simulink library "DAVS_lib"  (R2022b)
settings: Solver=VariableStepAuto  StartTime=0.0  StopTime=10.0  RelTol=1e-3
undefined symbols (not defined in the file): c0_ne, c0_pe, c_max_ne, c_max_pe, D_ne, D_pe, F, k, N_a_ne, N_a_pe, R_ne, R_pe
libraries: fl_lib x60, nesl_utility x60
(part 2 of 2)

== system DAVS_lib/DAVS/c_surf_ne/V(3)1/c(3) ==
  I(3) : Inport
  n : Inport  Port=2
  Divide : Product  Inputs=*/
  Gain : Gain  Gain=F
  Integrator : Integrator  InitialCondition=c0_ne
  Subsystem1 : Subsystem
  c(3) : Outport
  wires:
  Subsystem1/1(dV(n)1) -> Gain/1
  n/1 -> Subsystem1/1(n1)
  Integrator/1 -> c(3)/1
  Divide/1 -> Integrator/1
  Gain/1 -> Divide/2
  I(3)/1 -> Divide/1

== system DAVS_lib/DAVS/c_surf_ne/V(4)1/I(4) ==
  I_bar(3) : Inport
  I_bar(4) : Inport  Port=2
  Sum : Sum  Inputs=|-+|
  I(4) : Outport
  wires:
  I_bar(4)/1 -> Sum/1
  I_bar(3)/1 -> Sum/2
  Sum/1 -> I(4)/1

== system DAVS_lib/DAVS/c_surf_ne/V(4)1/Subsystem1 ==
  n : Inport
  Constant : Constant  Value=2
  Constant1 : Constant  Value=10
  Divide : Product  Inputs=*/
  Gain : Gain  Gain=k
  Gain1 : Gain  Gain=4*pi*R_ne*D_ne
  Math Function : Math  Operator=pow
  Rd : Outport
  wires:
  Constant1/1 -> Gain/1
  Divide/1 -> Rd/1
  Math Function/1 -> Gain1/1
  Gain1/1 -> Divide/2
  Constant/1 -> Math Function/2
  Gain/1 -> Divide/1
  n/1 -> Math Function/1

== system DAVS_lib/DAVS/c_surf_ne/V(4)1/V(4) ==
  c(4) : Inport
  Gain : Gain  Gain=k*F
  V(4) : Outport
  wires:
  c(4)/1 -> Gain/1
  Gain/1 -> V(4)/1

== system DAVS_lib/DAVS/c_surf_ne/V(4)1/c(4) ==
  I(4) : Inport
  n : Inport  Port=2
  Divide : Product  Inputs=*/
  Gain : Gain  Gain=F
  Integrator : Integrator  InitialCondition=c0_ne
  Subsystem1 : Subsystem
  c(4) : Outport
  wires:
  Subsystem1/1(dV(n)1) -> Gain/1
  n/1 -> Subsystem1/1(n1)
  I(4)/1 -> Divide/1
  Gain/1 -> Divide/2
  Divide/1 -> Integrator/1
  Integrator/1 -> c(4)/1

== system DAVS_lib/DAVS/c_surf_ne/V(5)1/I(n) ==
  I_bar(4) : Inport
  I_bar(5) : Inport  Port=2
  Sum : Sum  Inputs=|-+|
  I(5) : Outport
  wires:
  Sum/1 -> I(5)/1
  I_bar(4)/1 -> Sum/2
  I_bar(5)/1 -> Sum/1

== system DAVS_lib/DAVS/c_surf_ne/V(5)1/Subsystem1 ==
  n : Inport
  Constant : Constant  Value=2
  Constant1 : Constant  Value=10
  Divide : Product  Inputs=*/
  Gain : Gain  Gain=k
  Gain1 : Gain  Gain=4*pi*R_ne*D_ne
  Math Function : Math  Operator=pow
  Rd : Outport
  wires:
  Constant1/1 -> Gain/1
  Divide/1 -> Rd/1
  Math Function/1 -> Gain1/1
  Gain1/1 -> Divide/2
  Constant/1 -> Math Function/2
  Gain/1 -> Divide/1
  n/1 -> Math Function/1

== system DAVS_lib/DAVS/c_surf_ne/V(5)1/V(5) ==
  c(5) : Inport
  Gain : Gain  Gain=k*F
  V(5) : Outport
  wires:
  Gain/1 -> V(5)/1
  c(5)/1 -> Gain/1

== system DAVS_lib/DAVS/c_surf_ne/V(5)1/c(5) ==
  I(5) : Inport
  n : Inport  Port=2
  Divide : Product  Inputs=*/
  Gain : Gain  Gain=F
  Integrator : Integrator  InitialCondition=c0_ne
  Subsystem1 : Subsystem
  c(5) : Outport
  wires:
  Subsystem1/1(dV(n)1) -> Gain/1
  n/1 -> Subsystem1/1(n1)
  Integrator/1 -> c(5)/1
  Divide/1 -> Integrator/1
  Gain/1 -> Divide/2
  I(5)/1 -> Divide/1

== system DAVS_lib/DAVS/c_surf_ne/V(6)1/I(6) ==
  I_bar(6) : Inport
  I_bar(5) : Inport  Port=2
  Sum : Sum  Inputs=|-+|
  I(6) : Outport
  wires:
  I_bar(5)/1 -> Sum/1
  I_bar(6)/1 -> Sum/2
  Sum/1 -> I(6)/1

== system DAVS_lib/DAVS/c_surf_ne/V(6)1/Subsystem1 ==
  n : Inport
  Constant : Constant  Value=2
  Constant1 : Constant  Value=10
  Divide : Product  Inputs=*/
  Gain : Gain  Gain=k
  Gain1 : Gain  Gain=4*pi*R_ne*D_ne
  Math Function : Math  Operator=pow
  Rd : Outport
  wires:
  Constant1/1 -> Gain/1
  Divide/1 -> Rd/1
  Math Function/1 -> Gain1/1
  Gain1/1 -> Divide/2
  Constant/1 -> Math Function/2
  Gain/1 -> Divide/1
  n/1 -> Math Function/1

== system DAVS_lib/DAVS/c_surf_ne/V(6)1/V(6) ==
  c(6) : Inport
  Gain : Gain  Gain=k*F
  V(6) : Outport
  wires:
  c(6)/1 -> Gain/1
  Gain/1 -> V(6)/1

== system DAVS_lib/DAVS/c_surf_ne/V(6)1/c(6) ==
  I(6) : Inport
  n : Inport  Port=2
  Divide : Product  Inputs=*/
  Gain : Gain  Gain=F
  Integrator : Integrator  InitialCondition=c0_ne
  Subsystem1 : Subsystem
  c(6) : Outport
  wires:
  n/1 -> Subsystem1/1(n1)
  Subsystem1/1(dV(n)1) -> Gain/1
  I(6)/1 -> Divide/1
  Gain/1 -> Divide/2
  Divide/1 -> Integrator/1
  Integrator/1 -> c(6)/1

== system DAVS_lib/DAVS/c_surf_ne/V(7)1/I(7) ==
  I_bar(6) : Inport
  I_bar(7) : Inport  Port=2
  Sum : Sum  Inputs=|-+|
  I(7) : Outport
  wires:
  Sum/1 -> I(7)/1
  I_bar(6)/1 -> Sum/2
  I_bar(7)/1 -> Sum/1

== system DAVS_lib/DAVS/c_surf_ne/V(7)1/Subsystem1 ==
  n : Inport
  Constant : Constant  Value=2
  Constant1 : Constant  Value=10
  Divide : Product  Inputs=*/
  Gain : Gain  Gain=k
  Gain1 : Gain  Gain=4*pi*R_ne*D_ne
  Math Function : Math  Operator=pow
  Rd : Outport
  wires:
  Constant1/1 -> Gain/1
  Divide/1 -> Rd/1
  Math Function/1 -> Gain1/1
  Gain1/1 -> Divide/2
  Constant/1 -> Math Function/2
  Gain/1 -> Divide/1
  n/1 -> Math Function/1

== system DAVS_lib/DAVS/c_surf_ne/V(7)1/V(7) ==
  c(7) : Inport
  Gain : Gain  Gain=k*F
  V(7) : Outport
  wires:
  Gain/1 -> V(7)/1
  c(7)/1 -> Gain/1

== system DAVS_lib/DAVS/c_surf_ne/V(7)1/c(7) ==
  I(7) : Inport
  n : Inport  Port=2
  Divide : Product  Inputs=*/
  Gain : Gain  Gain=F
  Integrator : Integrator  InitialCondition=c0_ne
  Subsystem : Subsystem
  c(7) : Outport
  wires:
  Subsystem/1(dV(n)1) -> Gain/1
  n/1 -> Subsystem/1(n1)
  Integrator/1 -> c(7)/1
  Divide/1 -> Integrator/1
  Gain/1 -> Divide/2
  I(7)/1 -> Divide/1

== system DAVS_lib/DAVS/c_surf_ne/V(8)1/I(8) ==
  I_bar(7) : Inport
  I_bar(8) : Inport  Port=2
  Sum : Sum  Inputs=|-+|
  I(8) : Outport
  wires:
  I_bar(8)/1 -> Sum/1
  I_bar(7)/1 -> Sum/2
  Sum/1 -> I(8)/1

== system DAVS_lib/DAVS/c_surf_ne/V(8)1/Subsystem1 ==
  n : Inport
  Constant : Constant  Value=2
  Constant1 : Constant  Value=10
  Divide : Product  Inputs=*/
  Gain : Gain  Gain=k
  Gain1 : Gain  Gain=4*pi*R_ne*D_ne
  Math Function : Math  Operator=pow
  Rd : Outport
  wires:
  Constant1/1 -> Gain/1
  Divide/1 -> Rd/1
  Math Function/1 -> Gain1/1
  Gain1/1 -> Divide/2
  Constant/1 -> Math Function/2
  Gain/1 -> Divide/1
  n/1 -> Math Function/1

== system DAVS_lib/DAVS/c_surf_ne/V(8)1/V(8) ==
  c(8) : Inport
  Gain : Gain  Gain=k*F
  V(8) : Outport
  wires:
  c(8)/1 -> Gain/1
  Gain/1 -> V(8)/1

== system DAVS_lib/DAVS/c_surf_ne/V(8)1/c(1) ==
  I(8) : Inport
  n : Inport  Port=2
  Divide : Product  Inputs=*/
  Gain : Gain  Gain=F
  Integrator : Integrator  InitialCondition=c0_ne
  Subsystem : Subsystem
  c(8) : Outport
  wires:
  n/1 -> Subsystem/1(n1)
  Subsystem/1(dV(n)1) -> Gain/1
  I(8)/1 -> Divide/1
  Gain/1 -> Divide/2
  Divide/1 -> Integrator/1
  Integrator/1 -> c(8)/1

== system DAVS_lib/DAVS/c_surf_ne/V(9)1/I(9) ==
  I_bar(8) : Inport
  I_bar(9) : Inport  Port=2
  Sum : Sum  Inputs=|-+|
  I(9) : Outport
  wires:
  Sum/1 -> I(9)/1
  I_bar(8)/1 -> Sum/2
  I_bar(9)/1 -> Sum/1

== system DAVS_lib/DAVS/c_surf_ne/V(9)1/Subsystem1 ==
  n : Inport
  Constant : Constant  Value=2
  Constant1 : Constant  Value=10
  Divide : Product  Inputs=*/
  Gain : Gain  Gain=k
  Gain1 : Gain  Gain=4*pi*R_ne*D_ne
  Math Function : Math  Operator=pow
  Rd : Outport
  wires:
  Constant1/1 -> Gain/1
  Divide/1 -> Rd/1
  Math Function/1 -> Gain1/1
  Gain1/1 -> Divide/2
  Constant/1 -> Math Function/2
  Gain/1 -> Divide/1
  n/1 -> Math Function/1

== system DAVS_lib/DAVS/c_surf_ne/V(9)1/V(9) ==
  c(9) : Inport
  Gain : Gain  Gain=k*F
  V(9) : Outport
  wires:
  Gain/1 -> V(9)/1
  c(9)/1 -> Gain/1

== system DAVS_lib/DAVS/c_surf_ne/V(9)1/c(9) ==
  I(9) : Inport
  n : Inport  Port=2
  Divide : Product  Inputs=*/
  Gain : Gain  Gain=F
  Integrator : Integrator  InitialCondition=c0_ne
  Subsystem : Subsystem
  c(9) : Outport
  wires:
  n/1 -> Subsystem/1(n1)
  Subsystem/1(dV(n)1) -> Gain/1
  Integrator/1 -> c(9)/1
  Divide/1 -> Integrator/1
  Gain/1 -> Divide/2
  I(9)/1 -> Divide/1

== system DAVS_lib/DAVS/c_surf_pe/V(1)/I(1) ==
  I_bar(0) : Inport
  I_bar(1) : Inport  Port=2
  Sum : Sum  Inputs=|-+|
  I(1) : Outport
  wires:
  I_bar(1)/1 -> Sum/1
  I_bar(0)/1 -> Sum/2
  Sum/1 -> I(1)/1

== system DAVS_lib/DAVS/c_surf_pe/V(1)/Subsystem1 ==
  n : Inport
  Constant : Constant  Value=2
  Constant1 : Constant  Value=10
  Divide : Product  Inputs=*/
  Gain : Gain  Gain=k
  Gain1 : Gain  Gain=4*pi*R_pe*D_pe
  Math Function : Math  Operator=pow
  Rd : Outport
  wires:
  n/1 -> Math Function/1
  Gain/1 -> Divide/1
  Constant/1 -> Math Function/2
  Gain1/1 -> Divide/2
  Math Function/1 -> Gain1/1
  Divide/1 -> Rd/1
  Constant1/1 -> Gain/1

== system DAVS_lib/DAVS/c_surf_pe/V(1)/V(1) ==
  c(1) : Inport
  Gain : Gain  Gain=k*F
  V(1) : Outport
  wires:
  c(1)/1 -> Gain/1
  Gain/1 -> V(1)/1

== system DAVS_lib/DAVS/c_surf_pe/V(1)/c(1) ==
  I(1) : Inport
  n : Inport  Port=2
  Divide : Product  Inputs=*/
  Gain : Gain  Gain=F
  Integrator : Integrator  InitialCondition=c0_pe
  dV : Subsystem
  c(1) : Outport
  wires:
  I(1)/1 -> Divide/1
  Gain/1 -> Divide/2
  Divide/1 -> Integrator/1
  Integrator/1 -> c(1)/1
  dV/1(dV(n)) -> Gain/1
  n/1 -> dV/1(n)

== system DAVS_lib/DAVS/c_surf_pe/V(10)/I(10) ==
  I_bar(9) : Inport
  I_bar(10) : Inport  Port=2
  Sum : Sum  Inputs=|-+|
  I(10) : Outport
  wires:
  Sum/1 -> I(10)/1
  I_bar(9)/1 -> Sum/2
  I_bar(10)/1 -> Sum/1

== system DAVS_lib/DAVS/c_surf_pe/V(10)/Subsystem1 ==
  n : Inport
  Constant : Constant  Value=2
  Constant1 : Constant  Value=10
  Divide : Product  Inputs=*/
  Gain : Gain  Gain=k
  Gain1 : Gain  Gain=4*pi*R_pe*D_pe
  Math Function : Math  Operator=pow
  Rd : Outport
  wires:
  n/1 -> Math Function/1
  Gain/1 -> Divide/1
  Constant/1 -> Math Function/2
  Gain1/1 -> Divide/2
  Math Function/1 -> Gain1/1
  Divide/1 -> Rd/1
  Constant1/1 -> Gain/1

== system DAVS_lib/DAVS/c_surf_pe/V(10)/V(10) ==
  c(10) : Inport
  Gain : Gain  Gain=k*F
  V(10) : Outport
  wires:
  Gain/1 -> V(10)/1
  c(10)/1 -> Gain/1

== system DAVS_lib/DAVS/c_surf_pe/V(10)/c(10) ==
  I(10) : Inport
  n : Inport  Port=2
  Divide : Product  Inputs=*/
  Gain : Gain  Gain=F
  Integrator : Integrator  InitialCondition=c0_pe
  Subsystem : Subsystem
  c(10) : Outport
  wires:
  Integrator/1 -> c(10)/1
  Divide/1 -> Integrator/1
  Gain/1 -> Divide/2
  I(10)/1 -> Divide/1
  n/1 -> Subsystem/1(n1)
  Subsystem/1(dV(n)1) -> Gain/1

== system DAVS_lib/DAVS/c_surf_pe/V(2)/I(2) ==
  I_bar(1) : Inport
  I_bar(2) : Inport  Port=2
  Sum : Sum  Inputs=|-+|
  I(2) : Outport
  wires:
  Sum/1 -> I(2)/1
  I_bar(1)/1 -> Sum/2
  I_bar(2)/1 -> Sum/1

== system DAVS_lib/DAVS/c_surf_pe/V(2)/Subsystem1 ==
  n : Inport
  Constant : Constant  Value=2
  Constant1 : Constant  Value=10
  Divide : Product  Inputs=*/
  Gain : Gain  Gain=k
  Gain1 : Gain  Gain=4*pi*R_pe*D_pe
  Math Function : Math  Operator=pow
  Rd : Outport
  wires:
  n/1 -> Math Function/1
  Gain/1 -> Divide/1
  Constant/1 -> Math Function/2
  Gain1/1 -> Divide/2
  Math Function/1 -> Gain1/1
  Divide/1 -> Rd/1
  Constant1/1 -> Gain/1

== system DAVS_lib/DAVS/c_surf_pe/V(2)/V(2) ==
  c(2) : Inport
  Gain : Gain  Gain=k*F
  V(2) : Outport
  wires:
  Gain/1 -> V(2)/1
  c(2)/1 -> Gain/1

== system DAVS_lib/DAVS/c_surf_pe/V(2)/c(2) ==
  I(2) : Inport
  n : Inport  Port=2
  Divide : Product  Inputs=*/
  Gain : Gain  Gain=F
  Integrator : Integrator  InitialCondition=c0_pe
  Subsystem : Subsystem
  c(2) : Outport
  wires:
  Integrator/1 -> c(2)/1
  Divide/1 -> Integrator/1
  Gain/1 -> Divide/2
  I(2)/1 -> Divide/1
  n/1 -> Subsystem/1(n1)
  Subsystem/1(dV(n)1) -> Gain/1

== system DAVS_lib/DAVS/c_surf_pe/V(3)/I(3) ==
  I_bar(2) : Inport
  I_bar(3) : Inport  Port=2
  Sum : Sum  Inputs=|-+|
  I(3) : Outport
  wires:
  I_bar(3)/1 -> Sum/1
  I_bar(2)/1 -> Sum/2
  Sum/1 -> I(3)/1

== system DAVS_lib/DAVS/c_surf_pe/V(3)/Subsystem1 ==
  n : Inport
  Constant : Constant  Value=2
  Constant1 : Constant  Value=10
  Divide : Product  Inputs=*/
  Gain : Gain  Gain=k
  Gain1 : Gain  Gain=4*pi*R_pe*D_pe
  Math Function : Math  Operator=pow
  Rd : Outport
  wires:
  n/1 -> Math Function/1
  Gain/1 -> Divide/1
  Constant/1 -> Math Function/2
  Gain1/1 -> Divide/2
  Math Function/1 -> Gain1/1
  Divide/1 -> Rd/1
  Constant1/1 -> Gain/1

== system DAVS_lib/DAVS/c_surf_pe/V(3)/V(3) ==
  c(3) : Inport
  Gain : Gain  Gain=k*F
  V(3) : Outport
  wires:
  c(3)/1 -> Gain/1
  Gain/1 -> V(3)/1

== system DAVS_lib/DAVS/c_surf_pe/V(3)/c(3) ==
  I(3) : Inport
  n : Inport  Port=2
  Divide : Product  Inputs=*/
  Gain : Gain  Gain=F
  Integrator : Integrator  InitialCondition=c0_pe
  Subsystem1 : Subsystem
  c(3) : Outport
  wires:
  I(3)/1 -> Divide/1
  Gain/1 -> Divide/2
  Divide/1 -> Integrator/1
  Integrator/1 -> c(3)/1
  n/1 -> Subsystem1/1(n1)
  Subsystem1/1(dV(n)1) -> Gain/1

== system DAVS_lib/DAVS/c_surf_pe/V(4)/I(4) ==
  I_bar(3) : Inport
  I_bar(4) : Inport  Port=2
  Sum : Sum  Inputs=|-+|
  I(4) : Outport
  wires:
  Sum/1 -> I(4)/1
  I_bar(3)/1 -> Sum/2
  I_bar(4)/1 -> Sum/1

== system DAVS_lib/DAVS/c_surf_pe/V(4)/Subsystem1 ==
  n : Inport
  Constant : Constant  Value=2
  Constant1 : Constant  Value=10
  Divide : Product  Inputs=*/
  Gain : Gain  Gain=k
  Gain1 : Gain  Gain=4*pi*R_pe*D_pe
  Math Function : Math  Operator=pow
  Rd : Outport
  wires:
  n/1 -> Math Function/1
  Gain/1 -> Divide/1
  Constant/1 -> Math Function/2
  Gain1/1 -> Divide/2
  Math Function/1 -> Gain1/1
  Divide/1 -> Rd/1
  Constant1/1 -> Gain/1

== system DAVS_lib/DAVS/c_surf_pe/V(4)/V(4) ==
  c(4) : Inport
  Gain : Gain  Gain=k*F
  V(4) : Outport
  wires:
  Gain/1 -> V(4)/1
  c(4)/1 -> Gain/1

== system DAVS_lib/DAVS/c_surf_pe/V(4)/c(4) ==
  I(4) : Inport
  n : Inport  Port=2
  Divide : Product  Inputs=*/
  Gain : Gain  Gain=F
  Integrator : Integrator  InitialCondition=c0_pe
  Subsystem1 : Subsystem
  c(4) : Outport
  wires:
  Integrator/1 -> c(4)/1
  Divide/1 -> Integrator/1
  Gain/1 -> Divide/2
  I(4)/1 -> Divide/1
  n/1 -> Subsystem1/1(n1)
  Subsystem1/1(dV(n)1) -> Gain/1

== system DAVS_lib/DAVS/c_surf_pe/V(5)/I(n) ==
  I_bar(4) : Inport
  I_bar(5) : Inport  Port=2
  Sum : Sum  Inputs=|-+|
  I(5) : Outport
  wires:
  I_bar(5)/1 -> Sum/1
  I_bar(4)/1 -> Sum/2
  Sum/1 -> I(5)/1

== system DAVS_lib/DAVS/c_surf_pe/V(5)/Subsystem1 ==
  n : Inport
  Constant : Constant  Value=2
  Constant1 : Constant  Value=10
  Divide : Product  Inputs=*/
  Gain : Gain  Gain=k
  Gain1 : Gain  Gain=4*pi*R_pe*D_pe
  Math Function : Math  Operator=pow
  Rd : Outport
  wires:
  n/1 -> Math Function/1
  Gain/1 -> Divide/1
  Constant/1 -> Math Function/2
  Gain1/1 -> Divide/2
  Math Function/1 -> Gain1/1
  Divide/1 -> Rd/1
  Constant1/1 -> Gain/1

== system DAVS_lib/DAVS/c_surf_pe/V(5)/V(5) ==
  c(5) : Inport
  Gain : Gain  Gain=k*F
  V(5) : Outport
  wires:
  c(5)/1 -> Gain/1
  Gain/1 -> V(5)/1

== system DAVS_lib/DAVS/c_surf_pe/V(5)/c(5) ==
  I(5) : Inport
  n : Inport  Port=2
  Divide : Product  Inputs=*/
  Gain : Gain  Gain=F
  Integrator : Integrator  InitialCondition=c0_pe
  Subsystem1 : Subsystem
  c(5) : Outport
  wires:
  I(5)/1 -> Divide/1
  Gain/1 -> Divide/2
  Divide/1 -> Integrator/1
  Integrator/1 -> c(5)/1
  n/1 -> Subsystem1/1(n1)
  Subsystem1/1(dV(n)1) -> Gain/1

== system DAVS_lib/DAVS/c_surf_pe/V(6)/I(6) ==
  I_bar(6) : Inport
  I_bar(5) : Inport  Port=2
  Sum : Sum  Inputs=|-+|
  I(6) : Outport
  wires:
  Sum/1 -> I(6)/1
  I_bar(6)/1 -> Sum/2
  I_bar(5)/1 -> Sum/1

== system DAVS_lib/DAVS/c_surf_pe/V(6)/Subsystem1 ==
  n : Inport
  Constant : Constant  Value=2
  Constant1 : Constant  Value=10
  Divide : Product  Inputs=*/
  Gain : Gain  Gain=k
  Gain1 : Gain  Gain=4*pi*R_pe*D_pe
  Math Function : Math  Operator=pow
  Rd : Outport
  wires:
  n/1 -> Math Function/1
  Gain/1 -> Divide/1
  Constant/1 -> Math Function/2
  Gain1/1 -> Divide/2
  Math Function/1 -> Gain1/1
  Divide/1 -> Rd/1
  Constant1/1 -> Gain/1

== system DAVS_lib/DAVS/c_surf_pe/V(6)/V(6) ==
  c(6) : Inport
  Gain : Gain  Gain=k*F
  V(6) : Outport
  wires:
  Gain/1 -> V(6)/1
  c(6)/1 -> Gain/1

== system DAVS_lib/DAVS/c_surf_pe/V(6)/c(6) ==
  I(6) : Inport
  n : Inport  Port=2
  Divide : Product  Inputs=*/
  Gain : Gain  Gain=F
  Integrator : Integrator  InitialCondition=c0_pe
  Subsystem1 : Subsystem
  c(6) : Outport
  wires:
  Integrator/1 -> c(6)/1
  Divide/1 -> Integrator/1
  Gain/1 -> Divide/2
  I(6)/1 -> Divide/1
  Subsystem1/1(dV(n)1) -> Gain/1
  n/1 -> Subsystem1/1(n1)

== system DAVS_lib/DAVS/c_surf_pe/V(7)/I(7) ==
  I_bar(6) : Inport
  I_bar(7) : Inport  Port=2
  Sum : Sum  Inputs=|-+|
  I(7) : Outport
  wires:
  I_bar(7)/1 -> Sum/1
  I_bar(6)/1 -> Sum/2
  Sum/1 -> I(7)/1

== system DAVS_lib/DAVS/c_surf_pe/V(7)/Subsystem1 ==
  n : Inport
  Constant : Constant  Value=2
  Constant1 : Constant  Value=10
  Divide : Product  Inputs=*/
  Gain : Gain  Gain=k
  Gain1 : Gain  Gain=4*pi*R_pe*D_pe
  Math Function : Math  Operator=pow
  Rd : Outport
  wires:
  n/1 -> Math Function/1
  Gain/1 -> Divide/1
  Constant/1 -> Math Function/2
  Gain1/1 -> Divide/2
  Math Function/1 -> Gain1/1
  Divide/1 -> Rd/1
  Constant1/1 -> Gain/1

== system DAVS_lib/DAVS/c_surf_pe/V(7)/V(7) ==
  c(7) : Inport
  Gain : Gain  Gain=k*F
  V(7) : Outport
  wires:
  c(7)/1 -> Gain/1
  Gain/1 -> V(7)/1

== system DAVS_lib/DAVS/c_surf_pe/V(7)/c(7) ==
  I(7) : Inport
  n : Inport  Port=2
  Divide : Product  Inputs=*/
  Gain : Gain  Gain=F
  Integrator : Integrator  InitialCondition=c0_pe
  Subsystem : Subsystem
  c(7) : Outport
  wires:
  I(7)/1 -> Divide/1
  Gain/1 -> Divide/2
  Divide/1 -> Integrator/1
  Integrator/1 -> c(7)/1
  n/1 -> Subsystem/1(n1)
  Subsystem/1(dV(n)1) -> Gain/1

== system DAVS_lib/DAVS/c_surf_pe/V(8)/I(8) ==
  I_bar(7) : Inport
  I_bar(8) : Inport  Port=2
  Sum : Sum  Inputs=|-+|
  I(8) : Outport
  wires:
  Sum/1 -> I(8)/1
  I_bar(7)/1 -> Sum/2
  I_bar(8)/1 -> Sum/1

== system DAVS_lib/DAVS/c_surf_pe/V(8)/Subsystem1 ==
  n : Inport
  Constant : Constant  Value=2
  Constant1 : Constant  Value=10
  Divide : Product  Inputs=*/
  Gain : Gain  Gain=k
  Gain1 : Gain  Gain=4*pi*R_pe*D_pe
  Math Function : Math  Operator=pow
  Rd : Outport
  wires:
  n/1 -> Math Function/1
  Gain/1 -> Divide/1
  Constant/1 -> Math Function/2
  Gain1/1 -> Divide/2
  Math Function/1 -> Gain1/1
  Divide/1 -> Rd/1
  Constant1/1 -> Gain/1

== system DAVS_lib/DAVS/c_surf_pe/V(8)/V(8) ==
  c(8) : Inport
  Gain : Gain  Gain=k*F
  V(8) : Outport
  wires:
  Gain/1 -> V(8)/1
  c(8)/1 -> Gain/1

== system DAVS_lib/DAVS/c_surf_pe/V(8)/c(1) ==
  I(8) : Inport
  n : Inport  Port=2
  Divide : Product  Inputs=*/
  Gain : Gain  Gain=F
  Integrator : Integrator  InitialCondition=c0_pe
  Subsystem : Subsystem
  c(8) : Outport
  wires:
  Integrator/1 -> c(8)/1
  Divide/1 -> Integrator/1
  Gain/1 -> Divide/2
  I(8)/1 -> Divide/1
  Subsystem/1(dV(n)1) -> Gain/1
  n/1 -> Subsystem/1(n1)

== system DAVS_lib/DAVS/c_surf_pe/V(9)/I(9) ==
  I_bar(8) : Inport
  I_bar(9) : Inport  Port=2
  Sum : Sum  Inputs=|-+|
  I(9) : Outport
  wires:
  I_bar(9)/1 -> Sum/1
  I_bar(8)/1 -> Sum/2
  Sum/1 -> I(9)/1

== system DAVS_lib/DAVS/c_surf_pe/V(9)/Subsystem1 ==
  n : Inport
  Constant : Constant  Value=2
  Constant1 : Constant  Value=10
  Divide : Product  Inputs=*/
  Gain : Gain  Gain=k
  Gain1 : Gain  Gain=4*pi*R_pe*D_pe
  Math Function : Math  Operator=pow
  Rd : Outport
  wires:
  n/1 -> Math Function/1
  Gain/1 -> Divide/1
  Constant/1 -> Math Function/2
  Gain1/1 -> Divide/2
  Math Function/1 -> Gain1/1
  Divide/1 -> Rd/1
  Constant1/1 -> Gain/1

== system DAVS_lib/DAVS/c_surf_pe/V(9)/V(9) ==
  c(9) : Inport
  Gain : Gain  Gain=k*F
  V(9) : Outport
  wires:
  c(9)/1 -> Gain/1
  Gain/1 -> V(9)/1

== system DAVS_lib/DAVS/c_surf_pe/V(9)/c(9) ==
  I(9) : Inport
  n : Inport  Port=2
  Divide : Product  Inputs=*/
  Gain : Gain  Gain=F
  Integrator : Integrator  InitialCondition=c0_pe
  Subsystem : Subsystem
  c(9) : Outport
  wires:
  I(9)/1 -> Divide/1
  Gain/1 -> Divide/2
  Divide/1 -> Integrator/1
  Integrator/1 -> c(9)/1
  Subsystem/1(dV(n)1) -> Gain/1
  n/1 -> Subsystem/1(n1)

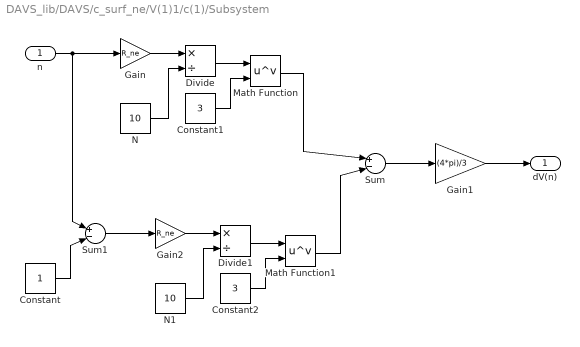
== system DAVS_lib/DAVS/c_surf_ne/V(1)1/c(1)/Subsystem ==
  n : Inport
  Constant : Constant
  Constant1 : Constant  Value=3
  Constant2 : Constant  Value=3
  Divide : Product  Inputs=*/
  Divide1 : Product  Inputs=*/
  Gain : Gain  Gain=R_ne
  Gain1 : Gain  Gain=(4*pi)/3
  Gain2 : Gain  Gain=R_ne
  Math Function : Math  Operator=pow
  Math Function1 : Math  Operator=pow
  N : Constant  Value=10
  N1 : Constant  Value=10
  Sum : Sum  Inputs=|+-|
  Sum1 : Sum  Inputs=|+-|
  dV(n) : Outport
  wires:
  Sum/1 -> Gain1/1
  Math Function1/1 -> Sum/2
  N1/1 -> Divide1/2
  Constant2/1 -> Math Function1/2
  Gain2/1 -> Divide1/1
  Divide1/1 -> Math Function1/1
  Sum1/1 -> Gain2/1
  Constant/1 -> Sum1/2
  Gain1/1 -> dV(n)/1
  Math Function/1 -> Sum/1
  Constant1/1 -> Math Function/2
  Divide/1 -> Math Function/1
  N/1 -> Divide/2
  Gain/1 -> Divide/1
  n/1 -> Gain/1, Sum1/1

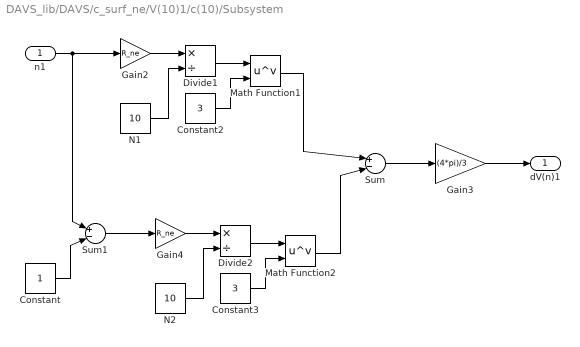
== system DAVS_lib/DAVS/c_surf_ne/V(10)1/c(10)/Subsystem ==
  n1 : Inport
  Constant : Constant
  Constant2 : Constant  Value=3
  Constant3 : Constant  Value=3
  Divide1 : Product  Inputs=*/
  Divide2 : Product  Inputs=*/
  Gain2 : Gain  Gain=R_ne
  Gain3 : Gain  Gain=(4*pi)/3
  Gain4 : Gain  Gain=R_ne
  Math Function1 : Math  Operator=pow
  Math Function2 : Math  Operator=pow
  N1 : Constant  Value=10
  N2 : Constant  Value=10
  Sum : Sum  Inputs=|+-|
  Sum1 : Sum  Inputs=|+-|
  dV(n)1 : Outport
  wires:
  Sum1/1 -> Gain4/1
  n1/1 -> Gain2/1, Sum1/1
  Divide1/1 -> Math Function1/1
  Math Function1/1 -> Sum/1
  Divide2/1 -> Math Function2/1
  Constant3/1 -> Math Function2/2
  N2/1 -> Divide2/2
  Sum/1 -> Gain3/1
  Gain4/1 -> Divide2/1
  Constant/1 -> Sum1/2
  Constant2/1 -> Math Function1/2
  N1/1 -> Divide1/2
  Gain2/1 -> Divide1/1
  Gain3/1 -> dV(n)1/1
  Math Function2/1 -> Sum/2

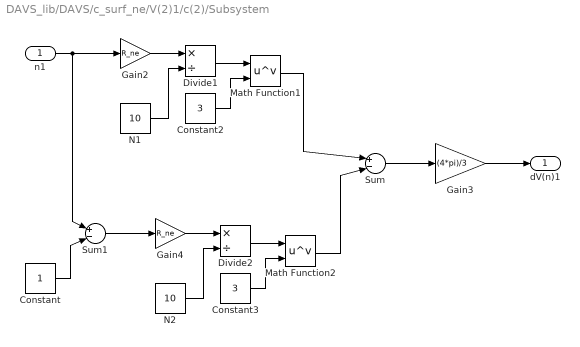
== system DAVS_lib/DAVS/c_surf_ne/V(2)1/c(2)/Subsystem ==
  n1 : Inport
  Constant : Constant
  Constant2 : Constant  Value=3
  Constant3 : Constant  Value=3
  Divide1 : Product  Inputs=*/
  Divide2 : Product  Inputs=*/
  Gain2 : Gain  Gain=R_ne
  Gain3 : Gain  Gain=(4*pi)/3
  Gain4 : Gain  Gain=R_ne
  Math Function1 : Math  Operator=pow
  Math Function2 : Math  Operator=pow
  N1 : Constant  Value=10
  N2 : Constant  Value=10
  Sum : Sum  Inputs=|+-|
  Sum1 : Sum  Inputs=|+-|
  dV(n)1 : Outport
  wires:
  Sum1/1 -> Gain4/1
  n1/1 -> Gain2/1, Sum1/1
  Divide1/1 -> Math Function1/1
  Math Function1/1 -> Sum/1
  Divide2/1 -> Math Function2/1
  Constant3/1 -> Math Function2/2
  N2/1 -> Divide2/2
  Sum/1 -> Gain3/1
  Gain4/1 -> Divide2/1
  Constant/1 -> Sum1/2
  Constant2/1 -> Math Function1/2
  N1/1 -> Divide1/2
  Gain2/1 -> Divide1/1
  Gain3/1 -> dV(n)1/1
  Math Function2/1 -> Sum/2

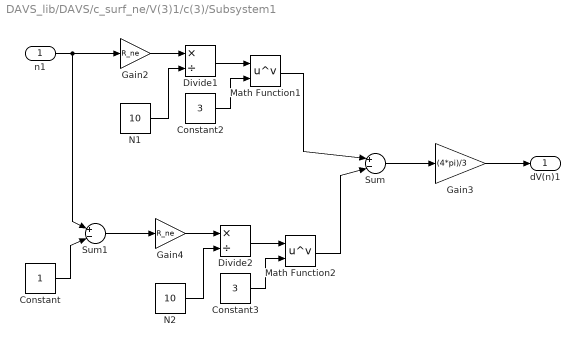
== system DAVS_lib/DAVS/c_surf_ne/V(3)1/c(3)/Subsystem1 ==
  n1 : Inport
  Constant : Constant
  Constant2 : Constant  Value=3
  Constant3 : Constant  Value=3
  Divide1 : Product  Inputs=*/
  Divide2 : Product  Inputs=*/
  Gain2 : Gain  Gain=R_ne
  Gain3 : Gain  Gain=(4*pi)/3
  Gain4 : Gain  Gain=R_ne
  Math Function1 : Math  Operator=pow
  Math Function2 : Math  Operator=pow
  N1 : Constant  Value=10
  N2 : Constant  Value=10
  Sum : Sum  Inputs=|+-|
  Sum1 : Sum  Inputs=|+-|
  dV(n)1 : Outport
  wires:
  Sum1/1 -> Gain4/1
  n1/1 -> Gain2/1, Sum1/1
  Divide1/1 -> Math Function1/1
  Math Function1/1 -> Sum/1
  Divide2/1 -> Math Function2/1
  Constant3/1 -> Math Function2/2
  N2/1 -> Divide2/2
  Sum/1 -> Gain3/1
  Gain4/1 -> Divide2/1
  Constant/1 -> Sum1/2
  Constant2/1 -> Math Function1/2
  N1/1 -> Divide1/2
  Gain2/1 -> Divide1/1
  Gain3/1 -> dV(n)1/1
  Math Function2/1 -> Sum/2

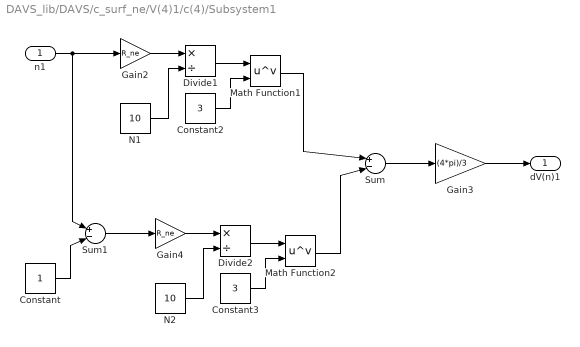
== system DAVS_lib/DAVS/c_surf_ne/V(4)1/c(4)/Subsystem1 ==
  n1 : Inport
  Constant : Constant
  Constant2 : Constant  Value=3
  Constant3 : Constant  Value=3
  Divide1 : Product  Inputs=*/
  Divide2 : Product  Inputs=*/
  Gain2 : Gain  Gain=R_ne
  Gain3 : Gain  Gain=(4*pi)/3
  Gain4 : Gain  Gain=R_ne
  Math Function1 : Math  Operator=pow
  Math Function2 : Math  Operator=pow
  N1 : Constant  Value=10
  N2 : Constant  Value=10
  Sum : Sum  Inputs=|+-|
  Sum1 : Sum  Inputs=|+-|
  dV(n)1 : Outport
  wires:
  Sum1/1 -> Gain4/1
  n1/1 -> Gain2/1, Sum1/1
  Divide1/1 -> Math Function1/1
  Math Function1/1 -> Sum/1
  Divide2/1 -> Math Function2/1
  Constant3/1 -> Math Function2/2
  N2/1 -> Divide2/2
  Sum/1 -> Gain3/1
  Gain4/1 -> Divide2/1
  Constant/1 -> Sum1/2
  Constant2/1 -> Math Function1/2
  N1/1 -> Divide1/2
  Gain2/1 -> Divide1/1
  Gain3/1 -> dV(n)1/1
  Math Function2/1 -> Sum/2

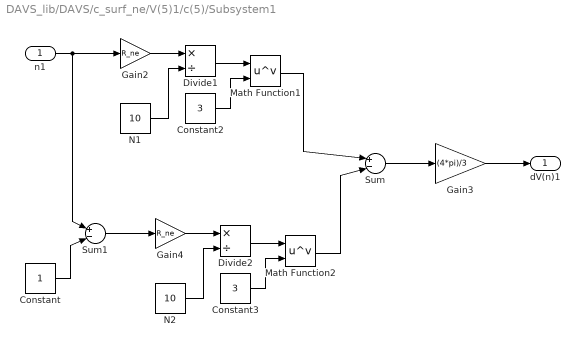
== system DAVS_lib/DAVS/c_surf_ne/V(5)1/c(5)/Subsystem1 ==
  n1 : Inport
  Constant : Constant
  Constant2 : Constant  Value=3
  Constant3 : Constant  Value=3
  Divide1 : Product  Inputs=*/
  Divide2 : Product  Inputs=*/
  Gain2 : Gain  Gain=R_ne
  Gain3 : Gain  Gain=(4*pi)/3
  Gain4 : Gain  Gain=R_ne
  Math Function1 : Math  Operator=pow
  Math Function2 : Math  Operator=pow
  N1 : Constant  Value=10
  N2 : Constant  Value=10
  Sum : Sum  Inputs=|+-|
  Sum1 : Sum  Inputs=|+-|
  dV(n)1 : Outport
  wires:
  Sum1/1 -> Gain4/1
  n1/1 -> Gain2/1, Sum1/1
  Divide1/1 -> Math Function1/1
  Math Function1/1 -> Sum/1
  Divide2/1 -> Math Function2/1
  Constant3/1 -> Math Function2/2
  N2/1 -> Divide2/2
  Sum/1 -> Gain3/1
  Gain4/1 -> Divide2/1
  Constant/1 -> Sum1/2
  Constant2/1 -> Math Function1/2
  N1/1 -> Divide1/2
  Gain2/1 -> Divide1/1
  Gain3/1 -> dV(n)1/1
  Math Function2/1 -> Sum/2

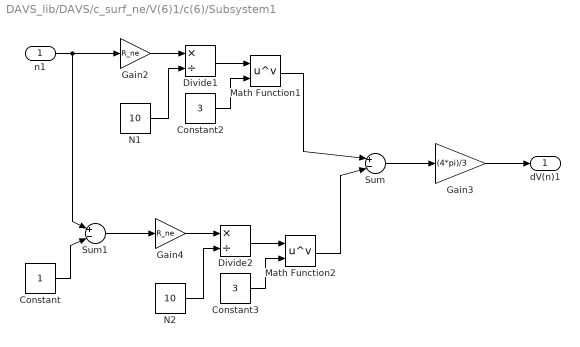
== system DAVS_lib/DAVS/c_surf_ne/V(6)1/c(6)/Subsystem1 ==
  n1 : Inport
  Constant : Constant
  Constant2 : Constant  Value=3
  Constant3 : Constant  Value=3
  Divide1 : Product  Inputs=*/
  Divide2 : Product  Inputs=*/
  Gain2 : Gain  Gain=R_ne
  Gain3 : Gain  Gain=(4*pi)/3
  Gain4 : Gain  Gain=R_ne
  Math Function1 : Math  Operator=pow
  Math Function2 : Math  Operator=pow
  N1 : Constant  Value=10
  N2 : Constant  Value=10
  Sum : Sum  Inputs=|+-|
  Sum1 : Sum  Inputs=|+-|
  dV(n)1 : Outport
  wires:
  Sum1/1 -> Gain4/1
  n1/1 -> Gain2/1, Sum1/1
  Divide1/1 -> Math Function1/1
  Math Function1/1 -> Sum/1
  Divide2/1 -> Math Function2/1
  Constant3/1 -> Math Function2/2
  N2/1 -> Divide2/2
  Sum/1 -> Gain3/1
  Gain4/1 -> Divide2/1
  Constant/1 -> Sum1/2
  Constant2/1 -> Math Function1/2
  N1/1 -> Divide1/2
  Gain2/1 -> Divide1/1
  Gain3/1 -> dV(n)1/1
  Math Function2/1 -> Sum/2

== system DAVS_lib/DAVS/c_surf_ne/V(7)1/c(7)/Subsystem ==
  n1 : Inport
  Constant : Constant
  Constant2 : Constant  Value=3
  Constant3 : Constant  Value=3
  Divide1 : Product  Inputs=*/
  Divide2 : Product  Inputs=*/
  Gain2 : Gain  Gain=R_ne
  Gain3 : Gain  Gain=(4*pi)/3
  Gain4 : Gain  Gain=R_ne
  Math Function1 : Math  Operator=pow
  Math Function2 : Math  Operator=pow
  N1 : Constant  Value=10
  N2 : Constant  Value=10
  Sum : Sum  Inputs=|+-|
  Sum1 : Sum  Inputs=|+-|
  dV(n)1 : Outport
  wires:
  Sum1/1 -> Gain4/1
  n1/1 -> Gain2/1, Sum1/1
  Divide1/1 -> Math Function1/1
  Math Function1/1 -> Sum/1
  Divide2/1 -> Math Function2/1
  Constant3/1 -> Math Function2/2
  N2/1 -> Divide2/2
  Sum/1 -> Gain3/1
  Gain4/1 -> Divide2/1
  Constant/1 -> Sum1/2
  Constant2/1 -> Math Function1/2
  N1/1 -> Divide1/2
  Gain2/1 -> Divide1/1
  Gain3/1 -> dV(n)1/1
  Math Function2/1 -> Sum/2

== system DAVS_lib/DAVS/c_surf_ne/V(8)1/c(1)/Subsystem ==
  n1 : Inport
  Constant : Constant
  Constant2 : Constant  Value=3
  Constant3 : Constant  Value=3
  Divide1 : Product  Inputs=*/
  Divide2 : Product  Inputs=*/
  Gain2 : Gain  Gain=R_ne
  Gain3 : Gain  Gain=(4*pi)/3
  Gain4 : Gain  Gain=R_ne
  Math Function1 : Math  Operator=pow
  Math Function2 : Math  Operator=pow
  N1 : Constant  Value=10
  N2 : Constant  Value=10
  Sum : Sum  Inputs=|+-|
  Sum1 : Sum  Inputs=|+-|
  dV(n)1 : Outport
  wires:
  Sum1/1 -> Gain4/1
  n1/1 -> Gain2/1, Sum1/1
  Divide1/1 -> Math Function1/1
  Math Function1/1 -> Sum/1
  Divide2/1 -> Math Function2/1
  Constant3/1 -> Math Function2/2
  N2/1 -> Divide2/2
  Sum/1 -> Gain3/1
  Gain4/1 -> Divide2/1
  Constant/1 -> Sum1/2
  Constant2/1 -> Math Function1/2
  N1/1 -> Divide1/2
  Gain2/1 -> Divide1/1
  Gain3/1 -> dV(n)1/1
  Math Function2/1 -> Sum/2

== system DAVS_lib/DAVS/c_surf_ne/V(9)1/c(9)/Subsystem ==
  n1 : Inport
  Constant : Constant
  Constant2 : Constant  Value=3
  Constant3 : Constant  Value=3
  Divide1 : Product  Inputs=*/
  Divide2 : Product  Inputs=*/
  Gain2 : Gain  Gain=R_ne
  Gain3 : Gain  Gain=(4*pi)/3
  Gain4 : Gain  Gain=R_ne
  Math Function1 : Math  Operator=pow
  Math Function2 : Math  Operator=pow
  N1 : Constant  Value=10
  N2 : Constant  Value=10
  Sum : Sum  Inputs=|+-|
  Sum1 : Sum  Inputs=|+-|
  dV(n)1 : Outport
  wires:
  Sum1/1 -> Gain4/1
  n1/1 -> Gain2/1, Sum1/1
  Divide1/1 -> Math Function1/1
  Math Function1/1 -> Sum/1
  Divide2/1 -> Math Function2/1
  Constant3/1 -> Math Function2/2
  N2/1 -> Divide2/2
  Sum/1 -> Gain3/1
  Gain4/1 -> Divide2/1
  Constant/1 -> Sum1/2
  Constant2/1 -> Math Function1/2
  N1/1 -> Divide1/2
  Gain2/1 -> Divide1/1
  Gain3/1 -> dV(n)1/1
  Math Function2/1 -> Sum/2

== system DAVS_lib/DAVS/c_surf_pe/V(1)/c(1)/dV ==
  n : Inport
  Constant : Constant
  Constant1 : Constant  Value=3
  Constant2 : Constant  Value=3
  Divide : Product  Inputs=*/
  Divide1 : Product  Inputs=*/
  Gain : Gain  Gain=R_pe
  Gain1 : Gain  Gain=(4*pi)/3
  Gain2 : Gain  Gain=R_pe
  Math Function : Math  Operator=pow
  Math Function1 : Math  Operator=pow
  N : Constant  Value=10
  N1 : Constant  Value=10
  Sum : Sum  Inputs=|+-|
  Sum1 : Sum  Inputs=|+-|
  dV(n) : Outport
  wires:
  n/1 -> Sum1/1, Gain/1
  Gain/1 -> Divide/1
  N/1 -> Divide/2
  Divide/1 -> Math Function/1
  Constant1/1 -> Math Function/2
  Math Function/1 -> Sum/1
  Gain1/1 -> dV(n)/1
  Constant/1 -> Sum1/2
  Sum1/1 -> Gain2/1
  Divide1/1 -> Math Function1/1
  Gain2/1 -> Divide1/1
  Constant2/1 -> Math Function1/2
  N1/1 -> Divide1/2
  Math Function1/1 -> Sum/2
  Sum/1 -> Gain1/1

== system DAVS_lib/DAVS/c_surf_pe/V(10)/c(10)/Subsystem ==
  n1 : Inport
  Constant : Constant
  Constant2 : Constant  Value=3
  Constant3 : Constant  Value=3
  Divide1 : Product  Inputs=*/
  Divide2 : Product  Inputs=*/
  Gain2 : Gain  Gain=R_pe
  Gain3 : Gain  Gain=(4*pi)/3
  Gain4 : Gain  Gain=R_pe
  Math Function1 : Math  Operator=pow
  Math Function2 : Math  Operator=pow
  N1 : Constant  Value=10
  N2 : Constant  Value=10
  Sum : Sum  Inputs=|+-|
  Sum1 : Sum  Inputs=|+-|
  dV(n)1 : Outport
  wires:
  Math Function2/1 -> Sum/2
  Gain3/1 -> dV(n)1/1
  Gain2/1 -> Divide1/1
  N1/1 -> Divide1/2
  Constant2/1 -> Math Function1/2
  Constant/1 -> Sum1/2
  Gain4/1 -> Divide2/1
  Sum/1 -> Gain3/1
  N2/1 -> Divide2/2
  Constant3/1 -> Math Function2/2
  Divide2/1 -> Math Function2/1
  Math Function1/1 -> Sum/1
  Divide1/1 -> Math Function1/1
  n1/1 -> Sum1/1, Gain2/1
  Sum1/1 -> Gain4/1

== system DAVS_lib/DAVS/c_surf_pe/V(2)/c(2)/Subsystem ==
  n1 : Inport
  Constant : Constant
  Constant2 : Constant  Value=3
  Constant3 : Constant  Value=3
  Divide1 : Product  Inputs=*/
  Divide2 : Product  Inputs=*/
  Gain2 : Gain  Gain=R_pe
  Gain3 : Gain  Gain=(4*pi)/3
  Gain4 : Gain  Gain=R_pe
  Math Function1 : Math  Operator=pow
  Math Function2 : Math  Operator=pow
  N1 : Constant  Value=10
  N2 : Constant  Value=10
  Sum : Sum  Inputs=|+-|
  Sum1 : Sum  Inputs=|+-|
  dV(n)1 : Outport
  wires:
  Math Function2/1 -> Sum/2
  Gain3/1 -> dV(n)1/1
  Gain2/1 -> Divide1/1
  N1/1 -> Divide1/2
  Constant2/1 -> Math Function1/2
  Constant/1 -> Sum1/2
  Gain4/1 -> Divide2/1
  Sum/1 -> Gain3/1
  N2/1 -> Divide2/2
  Constant3/1 -> Math Function2/2
  Divide2/1 -> Math Function2/1
  Math Function1/1 -> Sum/1
  Divide1/1 -> Math Function1/1
  n1/1 -> Sum1/1, Gain2/1
  Sum1/1 -> Gain4/1

== system DAVS_lib/DAVS/c_surf_pe/V(3)/c(3)/Subsystem1 ==
  n1 : Inport
  Constant : Constant
  Constant2 : Constant  Value=3
  Constant3 : Constant  Value=3
  Divide1 : Product  Inputs=*/
  Divide2 : Product  Inputs=*/
  Gain2 : Gain  Gain=R_pe
  Gain3 : Gain  Gain=(4*pi)/3
  Gain4 : Gain  Gain=R_pe
  Math Function1 : Math  Operator=pow
  Math Function2 : Math  Operator=pow
  N1 : Constant  Value=10
  N2 : Constant  Value=10
  Sum : Sum  Inputs=|+-|
  Sum1 : Sum  Inputs=|+-|
  dV(n)1 : Outport
  wires:
  Math Function2/1 -> Sum/2
  Gain3/1 -> dV(n)1/1
  Gain2/1 -> Divide1/1
  N1/1 -> Divide1/2
  Constant2/1 -> Math Function1/2
  Constant/1 -> Sum1/2
  Gain4/1 -> Divide2/1
  Sum/1 -> Gain3/1
  N2/1 -> Divide2/2
  Constant3/1 -> Math Function2/2
  Divide2/1 -> Math Function2/1
  Math Function1/1 -> Sum/1
  Divide1/1 -> Math Function1/1
  n1/1 -> Sum1/1, Gain2/1
  Sum1/1 -> Gain4/1

== system DAVS_lib/DAVS/c_surf_pe/V(4)/c(4)/Subsystem1 ==
  n1 : Inport
  Constant : Constant
  Constant2 : Constant  Value=3
  Constant3 : Constant  Value=3
  Divide1 : Product  Inputs=*/
  Divide2 : Product  Inputs=*/
  Gain2 : Gain  Gain=R_pe
  Gain3 : Gain  Gain=(4*pi)/3
  Gain4 : Gain  Gain=R_pe
  Math Function1 : Math  Operator=pow
  Math Function2 : Math  Operator=pow
  N1 : Constant  Value=10
  N2 : Constant  Value=10
  Sum : Sum  Inputs=|+-|
  Sum1 : Sum  Inputs=|+-|
  dV(n)1 : Outport
  wires:
  Math Function2/1 -> Sum/2
  Gain3/1 -> dV(n)1/1
  Gain2/1 -> Divide1/1
  N1/1 -> Divide1/2
  Constant2/1 -> Math Function1/2
  Constant/1 -> Sum1/2
  Gain4/1 -> Divide2/1
  Sum/1 -> Gain3/1
  N2/1 -> Divide2/2
  Constant3/1 -> Math Function2/2
  Divide2/1 -> Math Function2/1
  Math Function1/1 -> Sum/1
  Divide1/1 -> Math Function1/1
  n1/1 -> Sum1/1, Gain2/1
  Sum1/1 -> Gain4/1

== system DAVS_lib/DAVS/c_surf_pe/V(5)/c(5)/Subsystem1 ==
  n1 : Inport
  Constant : Constant
  Constant2 : Constant  Value=3
  Constant3 : Constant  Value=3
  Divide1 : Product  Inputs=*/
  Divide2 : Product  Inputs=*/
  Gain2 : Gain  Gain=R_pe
  Gain3 : Gain  Gain=(4*pi)/3
  Gain4 : Gain  Gain=R_pe
  Math Function1 : Math  Operator=pow
  Math Function2 : Math  Operator=pow
  N1 : Constant  Value=10
  N2 : Constant  Value=10
  Sum : Sum  Inputs=|+-|
  Sum1 : Sum  Inputs=|+-|
  dV(n)1 : Outport
  wires:
  Math Function2/1 -> Sum/2
  Gain3/1 -> dV(n)1/1
  Gain2/1 -> Divide1/1
  N1/1 -> Divide1/2
  Constant2/1 -> Math Function1/2
  Constant/1 -> Sum1/2
  Gain4/1 -> Divide2/1
  Sum/1 -> Gain3/1
  N2/1 -> Divide2/2
  Constant3/1 -> Math Function2/2
  Divide2/1 -> Math Function2/1
  Math Function1/1 -> Sum/1
  Divide1/1 -> Math Function1/1
  n1/1 -> Sum1/1, Gain2/1
  Sum1/1 -> Gain4/1

== system DAVS_lib/DAVS/c_surf_pe/V(6)/c(6)/Subsystem1 ==
  n1 : Inport
  Constant : Constant
  Constant2 : Constant  Value=3
  Constant3 : Constant  Value=3
  Divide1 : Product  Inputs=*/
  Divide2 : Product  Inputs=*/
  Gain2 : Gain  Gain=R_pe
  Gain3 : Gain  Gain=(4*pi)/3
  Gain4 : Gain  Gain=R_pe
  Math Function1 : Math  Operator=pow
  Math Function2 : Math  Operator=pow
  N1 : Constant  Value=10
  N2 : Constant  Value=10
  Sum : Sum  Inputs=|+-|
  Sum1 : Sum  Inputs=|+-|
  dV(n)1 : Outport
  wires:
  Math Function2/1 -> Sum/2
  Gain3/1 -> dV(n)1/1
  Gain2/1 -> Divide1/1
  N1/1 -> Divide1/2
  Constant2/1 -> Math Function1/2
  Constant/1 -> Sum1/2
  Gain4/1 -> Divide2/1
  Sum/1 -> Gain3/1
  N2/1 -> Divide2/2
  Constant3/1 -> Math Function2/2
  Divide2/1 -> Math Function2/1
  Math Function1/1 -> Sum/1
  Divide1/1 -> Math Function1/1
  n1/1 -> Sum1/1, Gain2/1
  Sum1/1 -> Gain4/1

== system DAVS_lib/DAVS/c_surf_pe/V(7)/c(7)/Subsystem ==
  n1 : Inport
  Constant : Constant
  Constant2 : Constant  Value=3
  Constant3 : Constant  Value=3
  Divide1 : Product  Inputs=*/
  Divide2 : Product  Inputs=*/
  Gain2 : Gain  Gain=R_pe
  Gain3 : Gain  Gain=(4*pi)/3
  Gain4 : Gain  Gain=R_pe
  Math Function1 : Math  Operator=pow
  Math Function2 : Math  Operator=pow
  N1 : Constant  Value=10
  N2 : Constant  Value=10
  Sum : Sum  Inputs=|+-|
  Sum1 : Sum  Inputs=|+-|
  dV(n)1 : Outport
  wires:
  Math Function2/1 -> Sum/2
  Gain3/1 -> dV(n)1/1
  Gain2/1 -> Divide1/1
  N1/1 -> Divide1/2
  Constant2/1 -> Math Function1/2
  Constant/1 -> Sum1/2
  Gain4/1 -> Divide2/1
  Sum/1 -> Gain3/1
  N2/1 -> Divide2/2
  Constant3/1 -> Math Function2/2
  Divide2/1 -> Math Function2/1
  Math Function1/1 -> Sum/1
  Divide1/1 -> Math Function1/1
  n1/1 -> Sum1/1, Gain2/1
  Sum1/1 -> Gain4/1

== system DAVS_lib/DAVS/c_surf_pe/V(8)/c(1)/Subsystem ==
  n1 : Inport
  Constant : Constant
  Constant2 : Constant  Value=3
  Constant3 : Constant  Value=3
  Divide1 : Product  Inputs=*/
  Divide2 : Product  Inputs=*/
  Gain2 : Gain  Gain=R_pe
  Gain3 : Gain  Gain=(4*pi)/3
  Gain4 : Gain  Gain=R_pe
  Math Function1 : Math  Operator=pow
  Math Function2 : Math  Operator=pow
  N1 : Constant  Value=10
  N2 : Constant  Value=10
  Sum : Sum  Inputs=|+-|
  Sum1 : Sum  Inputs=|+-|
  dV(n)1 : Outport
  wires:
  Math Function2/1 -> Sum/2
  Gain3/1 -> dV(n)1/1
  Gain2/1 -> Divide1/1
  N1/1 -> Divide1/2
  Constant2/1 -> Math Function1/2
  Constant/1 -> Sum1/2
  Gain4/1 -> Divide2/1
  Sum/1 -> Gain3/1
  N2/1 -> Divide2/2
  Constant3/1 -> Math Function2/2
  Divide2/1 -> Math Function2/1
  Math Function1/1 -> Sum/1
  Divide1/1 -> Math Function1/1
  n1/1 -> Sum1/1, Gain2/1
  Sum1/1 -> Gain4/1

== system DAVS_lib/DAVS/c_surf_pe/V(9)/c(9)/Subsystem ==
  n1 : Inport
  Constant : Constant
  Constant2 : Constant  Value=3
  Constant3 : Constant  Value=3
  Divide1 : Product  Inputs=*/
  Divide2 : Product  Inputs=*/
  Gain2 : Gain  Gain=R_pe
  Gain3 : Gain  Gain=(4*pi)/3
  Gain4 : Gain  Gain=R_pe
  Math Function1 : Math  Operator=pow
  Math Function2 : Math  Operator=pow
  N1 : Constant  Value=10
  N2 : Constant  Value=10
  Sum : Sum  Inputs=|+-|
  Sum1 : Sum  Inputs=|+-|
  dV(n)1 : Outport
  wires:
  Math Function2/1 -> Sum/2
  Gain3/1 -> dV(n)1/1
  Gain2/1 -> Divide1/1
  N1/1 -> Divide1/2
  Constant2/1 -> Math Function1/2
  Constant/1 -> Sum1/2
  Gain4/1 -> Divide2/1
  Sum/1 -> Gain3/1
  N2/1 -> Divide2/2
  Constant3/1 -> Math Function2/2
  Divide2/1 -> Math Function2/1
  Math Function1/1 -> Sum/1
  Divide1/1 -> Math Function1/1
  n1/1 -> Sum1/1, Gain2/1
  Sum1/1 -> Gain4/1

== matlab function DAVS_lib/DAVS/I_app/I_app_pe ==
  data: currentTime input; signal output; I_app input
function signal = fcn(currentTime, I_app)
    % Define time intervals
    t1 = 1740;    % Duration of first signal
    t2 = 3600;    % Duration of second signal
    t3 = 1020;    % Duration of third signal
    t4 = 3624;    % Duration of fourth signal

    % Generate signal based on current time
    if currentTime <= t1
        signal = -I_app;
    elseif currentTime <= t1 + t2
        signal = 0;
    elseif currentTime <= t1 + t2 + t3
        signal = I_app;
    elseif currentTime <= t1 + t2 + t3 + t4
        signal = 0;
    else
        signal = 0;  % Default value for any other time
    end
end

== matlab function DAVS_lib/DAVS/I_app/I_app_ne ==
  data: currentTime input; signal output; I_app input
function signal = fcn(currentTime, I_app)
    % Define time intervals
    t1 = 1740;    % Duration of first signal
    t2 = 3600;    % Duration of second signal
    t3 = 1020;    % Duration of third signal
    t4 = 3624;    % Duration of fourth signal

    % Generate signal based on current time
    if currentTime <= t1
        signal = I_app;
    elseif currentTime <= t1 + t2
        signal = 0;
    elseif currentTime <= t1 + t2 + t3
        signal = -I_app;
    elseif currentTime <= t1 + t2 + t3 + t4
        signal = 0;
    else
        signal = 0;  % Default value for any other time
    end
end
